simulink library "SAMPLE_systems"  (R2019b)
settings: Solver=VariableStepAuto  StartTime=0.0  StopTime=10.0  RelTol=1e-3  EnableMultiTasking=on
undefined symbols (not defined in the file): I, M, omega0, orbit, q0, q_gen, zq
libraries: DQ_SR_LIB_SIM x3, Filters x2, aerolibutil x1
settings Model: Creator=rivolta  LastModifiedBy=AurelianoRivolta
settings DataIOCC: LimitDataPoints=on  ReturnWorkspaceOutputs=off
settings OptimizationCC: LifeSpan=inf
settings DebuggingCC: AllowSymbolicDim=off  SFUnexpectedBacktrackingDiag=warning  SFNoUnconditionalDefaultTransitionDiag=warning  SFExecutionAtInitializationDiag=none  ArithmeticOperatorsInVariantConditions=warning
settings ModelReferenceCC: PropagateSignalLabelsOutOfModel=off
settings SFSimCC: SimUseLocalCustomCode=off  CustomCodeUndefinedFunction=UseInterfaceOnly
settings RTWCC: RTWUseLocalCustomCode=off
settings CodeAppCC: StateflowObjectComments=on
settings GRTTargetCC: TargetLangStandard=C89/C90 (ANSI)
settings ConfigComp: CovMetricSettings=dw  CovHtmlReporting=on  CovSaveCumulativeToWorkspaceVar=on  CovSaveSingleToWorkspaceVar=on  CovExternalEMLEnable=off

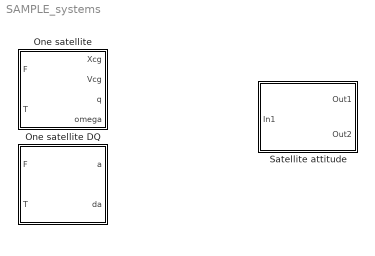
== system SAMPLE_systems ==
  One satellite : Subsystem  mask{M=100, I=[1;1;1]*100, a=1e8, ecc=0.2, incl=7, RAAN=6, omega=0, theta=0, q0=q_gen('x',pi/4), omega_b=[0;0;1]*1e-5*1, isin=off}
      mask prompts: M "Mass"; I "Inertia"; a "Semimajor axis [m]"; ecc "Eccentricity"; incl "Inclination"; omega "Pericenter anomaly"; theta "True anomaly"; q0 "Quaternion"; omega_b "Angular velocity"; isin "Inertial"
      mask init:
      | % add mass
      | II = [I;M];
      | 
      | % get position and velocity
      | mu=3.986*10^5*1e9;
      | 
      | radius = a*(1-ecc^2)/(1+ecc*cos(theta));
      | velocity = sqrt(mu/a)*(1+ecc*sin(theta));
      | 
      | R = angle2dcm(RAAN,incl,omega,'zxz');
      | 
      | Xcg=radius*R*[cos(theta);sin(theta);0];
      | Vcg=velocity*R*[-sin(theta);cos(theta);0];
      | 
      | XCG0=[Vcg;Xcg];
      | 
      | % get attitude (note: inertial w.r.t. body seems switched. 
      | % The input dq for the function is opposite, therefore the two systems are
      | % switched)
      | 
      | if isin == 0
      |     dq0=.5*crossqm([omega_b;0])*q0;
      | else
      |     dq0=.5*crossqp([omega_b;0])*q0;
      | end
      mask DialogControl Container3 Prompt: Mass properties
      mask DialogControl Container4 Prompt: Orbit
      mask DialogControl Container5 Prompt: Attitude
      mask Display:
      | port_label('input',1,'F_b','interpreter','tex')
      | port_label('input',2,'T_b','interpreter','tex')
      | port_label('output',1,'X_{cg}','interpreter','tex')
      | port_label('output',2,'V_{cg}','interpreter','tex')
      | port_label('output',3,'q','interpreter','tex')
      | port_label('output',4,'\omega_{b}','interpreter','tex')
      | fprintf('single\nsatellite')
  One satellite DQ : Subsystem  mask{M=M, I=I, a=orbit.a, ecc=orbit.e, incl=orbit.i, RAAN=orbit.RAAN, omega=orbit.omega, theta=orbit.theta, q0=q0, omega_b=omega0, isin=off}
      mask prompts: M "Mass"; I "Inertia"; a "Semimajor axis [m]"; ecc "Eccentricity"; incl "Inclination"; omega "Pericenter anomaly"; theta "True anomaly"; q0 "Quaternion"; omega_b "Angular velocity"; isin "Inertial"
      mask init: same as SAMPLE_systems/One satellite
      mask DialogControl Container3 Prompt: Mass properties
      mask DialogControl Container4 Prompt: Orbit
      mask DialogControl Container5 Prompt: Attitude
      mask Display:
      | port_label('input',1,'F_b','interpreter','tex')
      | port_label('input',2,'T_b','interpreter','tex')
      | port_label('output',1,'a','interpreter','tex')
      | port_label('output',2,'da','interpreter','tex')
      | fprintf('single\nsatellite')
  Satellite attitude : Subsystem  mask{omega0=rand(3,1), I=diag(100*[1;1;1]), q0=zq}
      mask prompts: omega0 "Initial angular velocity"; I "Inertia tensor"; q0 "Initial attitude"
      mask Display:
      | fprintf('Q-attitude')
      | port_label('input',1,'u')
      | port_label('output',1,'\omega_b','interpreter','tex')
      | port_label('output',2,'q')

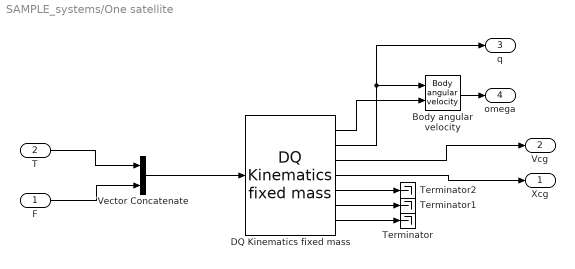
== system SAMPLE_systems/One satellite ==
  F : Inport
  T : Inport  Port=2
  Body angular velocity : DQ_SR_LIB_SIM/Utilities/Body  angular velocity
  DQ Kinematics fixed mass : DQ_SR_LIB_SIM/DQ Kinematics fixed mass  dynfun='onesat_S'  Gswitch=ECI gravity force  n_bodies=2  n_var0=5  n_ext=7  q_norm_in=[1:4]'  NORMONOFF=on  II=II  X0=[dq0;q0]  XCG0=XCG0  UPPERSAT=Inf  LOWERSAT=-Inf
  Terminator : Terminator
  Terminator1 : Terminator
  Terminator2 : Terminator
  Vector Concatenate : Concatenate
  Xcg : Outport
  Vcg : Outport  Port=2
  q : Outport  Port=3
  omega : Outport  Port=4
  wires:
  DQ Kinematics fixed mass/6 -> Terminator1/1
  DQ Kinematics fixed mass/5 -> Terminator2/1
  F/1 -> Vector Concatenate/2
  T/1 -> Vector Concatenate/1
  Vector Concatenate/1 -> DQ Kinematics fixed mass/1
  DQ Kinematics fixed mass/2 -> q/1, Body angular velocity/1
  DQ Kinematics fixed mass/1 -> Body angular velocity/2
  Body angular velocity/1 -> omega/1
  DQ Kinematics fixed mass/4 -> Xcg/1
  DQ Kinematics fixed mass/7 -> Terminator/1
  DQ Kinematics fixed mass/3 -> Vcg/1

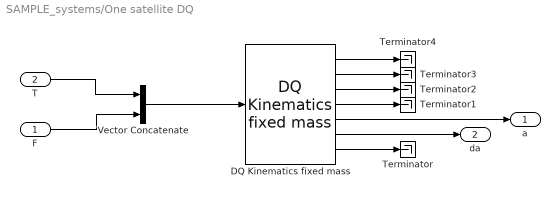
== system SAMPLE_systems/One satellite DQ ==
  F : Inport
  T : Inport  Port=2
  DQ Kinematics fixed mass : DQ_SR_LIB_SIM/DQ Kinematics fixed mass  dynfun='onesat_S'  Gswitch=ECI gravity force  n_bodies=2  n_var0=5  n_ext=7  q_norm_in=[1:4]'  NORMONOFF=on  II=II  X0=[dq0;q0]  XCG0=XCG0  UPPERSAT=Inf  LOWERSAT=-Inf
  Terminator{,1..4} (5 alike) : Terminator
  Vector Concatenate : Concatenate
  a : Outport
  da : Outport  Port=2
  wires:
  DQ Kinematics fixed mass/1 -> Terminator4/1
  DQ Kinematics fixed mass/2 -> Terminator3/1
  DQ Kinematics fixed mass/3 -> Terminator2/1
  DQ Kinematics fixed mass/4 -> Terminator1/1
  DQ Kinematics fixed mass/6 -> da/1
  DQ Kinematics fixed mass/5 -> a/1
  F/1 -> Vector Concatenate/2
  T/1 -> Vector Concatenate/1
  Vector Concatenate/1 -> DQ Kinematics fixed mass/1
  DQ Kinematics fixed mass/7 -> Terminator/1

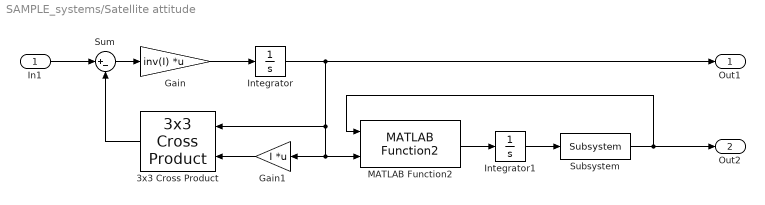
== system SAMPLE_systems/Satellite attitude ==
  In1 : Inport
  3x3 Cross Product : aerolibutil/3x3 Cross Product
      settings: SourceProductName=Aerospace Blockset  SourceProductBaseCode=AE
  Gain : Gain  Gain=inv(I)  Multiplication=Matrix(K*u)
  Gain1 : Gain  Gain=I  Multiplication=Matrix(K*u)
  Integrator : Integrator  InitialCondition=omega0
  Integrator1 : Integrator  InitialCondition=q0
  MATLAB Function2 : Filters/Non Linear Complementary Attitude filter/MATLAB Function2
  Subsystem : Filters/Non Linear Complementary Attitude filter/Subsystem  SystemSampleTime=-1
  Sum : Sum  Inputs=|+-
  Out1 : Outport
  Out2 : Outport  Port=2
  wires:
  3x3 Cross Product/1 -> Sum/2
  In1/1 -> Sum/1
  Sum/1 -> Gain/1
  Subsystem/1 -> Out2/1, MATLAB Function2/1
  Integrator1/1 -> Subsystem/1
  Gain/1 -> Integrator/1
  Integrator/1 -> Out1/1, MATLAB Function2/2, Gain1/1, 3x3 Cross Product/1
  Gain1/1 -> 3x3 Cross Product/2
  MATLAB Function2/1 -> Integrator1/1
